simulink model "sfcndemo_matadd"  (Simulink 6.0)
settings: Solver=FixedStepDiscrete  StartTime=0.0  StopTime=10.0  RelTol=1e-3
settings Model: Creator=The MathWorks Inc.  LastModifiedBy=batserve  ExtModeAutoUpdateStatusClock=off
settings DataIOCC: SaveOutput=off  OutputSaveName=y1,y2,y3,y4
settings OptimizationCC: BlockReduction=off  BooleanDataType=off
settings DebuggingCC: CheckExecutionContextPreStartOutputMsg=on  CheckExecutionContextRuntimeOutputMsg=on  SolverPrmCheckMsg=none
settings HardwareCC: TargetUnknown=on

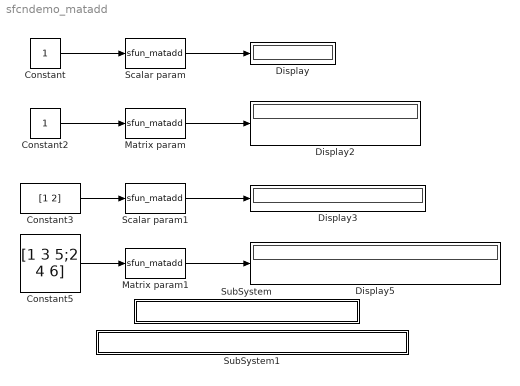
== system sfcndemo_matadd ==
  Constant : Constant  VectorParams1D=off
  Constant2 : Constant  VectorParams1D=off
  Constant3 : Constant  Value=[1 2]  VectorParams1D=off
  Constant5 : Constant  Value=[1 3 5;2 4 6]  VectorParams1D=off
  Display{,2..3,5} (4 alike) : Display
  Matrix param : S-Function  FunctionName=sfun_matadd  Parameters=Operand  mask(Matrix add){Operand=[1 3; 2 4]}
      mask prompts: Operand "Operand 1:"
      settings: AttributesFormatString=Param = %<Operand>
      mask Display: disp('Matrix\n Add ')
  Matrix param1 : S-Function  FunctionName=sfun_matadd  Parameters=Operand  mask(Matrix add){Operand=[1 3 5;2 4 6]}
      mask prompts: Operand "Operand 1:"
      settings: AttributesFormatString=Param = %<Operand>
      mask Display: disp('Matrix\n Add ')
  Scalar param : S-Function  FunctionName=sfun_matadd  Parameters=Operand  mask(Matrix add){Operand=1}
      mask prompts: Operand "Operand 1:"
      settings: AttributesFormatString=Param = %<Operand>
      mask Display: disp('Matrix\n Add ')
  Scalar param1 : S-Function  FunctionName=sfun_matadd  Parameters=Operand  mask(Matrix add){Operand=1}
      mask prompts: Operand "Operand 1:"
      settings: AttributesFormatString=Param = %<Operand>
      mask Display: disp('Matrix\n Add ')
  SubSystem : Subsystem  PropExecContextAcrossSSBoundary=on
      settings: OpenFcn=edit(fullfile(matlabroot,'simulink','src','sfun_matadd.c'))
      mask Display: disp('matlabroot\simulink\src\sfun_matadd.c');
  SubSystem1 : Subsystem  PropExecContextAcrossSSBoundary=on
      settings: OpenFcn=edit(fullfile(matlabroot,'toolbox','simulink','blocks','tlc_c','sfun_matadd.tlc'))
      mask Display: disp('matlabroot\toolbox\simulink\blocks\tlc_c\sfun_matadd.tlc');
  wires:
  Constant/1 -> Scalar param/1
  Scalar param/1 -> Display/1
  Constant2/1 -> Matrix param/1
  Matrix param/1 -> Display2/1
  Constant3/1 -> Scalar param1/1
  Scalar param1/1 -> Display3/1
  Constant5/1 -> Matrix param1/1
  Matrix param1/1 -> Display5/1

== system sfcndemo_matadd/SubSystem ==

== system sfcndemo_matadd/SubSystem1 ==
